simulink model "hiratsuka_dampa_1DOF"  (R2020a)
settings: Solver=ode4  StartTime=0.0  StopTime=10.0  FixedStep=0.002  RelTol=1e-3
values from neighbouring files (symbols this model uses):
  A = 1    [bode_hiratsuka_damper.m]    (also in exp_dampa.m = 0.007; mf_dampa_1DOF.m = 0.003; mf_feedback_relative.m = 0.003; mf_nonlinear_relative.m = 0.01)
  Aor = 0.1*10^-6    (= 1e-07)    [bode_hiratsuka_damper.m]    (also in exp_dampa.m; mf_dampa_1DOF.m; mf_feedback_relative.m; mf_nonlinear_relative.m)
  Ap = (32.50*0.001)^2*pi/4    (= 0.000829576810089)    [bode_hiratsuka_damper.m]    (also in exp_dampa.m; mf_dampa_1DOF.m; mf_feedback_relative.m; mf_nonlinear_relative.m)
  Cor = 0.8    [bode_hiratsuka_damper.m]    (also in exp_dampa.m; mf_dampa_1DOF.m; mf_feedback_relative.m; mf_nonlinear_relative.m)
  Hz = wv(k)    [bode_hiratsuka_damper.m]    (also in exp_dampa.m = 18.8495559215; mf_dampa_1DOF.m = 6.28318530718; mf_feedback_relative.m = 6.28318530718; mf_nonlinear_relative.m = 6.28318530718)
  k1 = 2200    [mf_dampa_1DOF.m]    (also in mf_feedback_relative.m; mf_nonlinear_relative.m; mf_with_P.m; mf_with_Pm.m)
  k2 = 405    [mf_dampa_1DOF.m]    (also in mf_feedback_relative.m; mf_nonlinear_relative.m; mf_with_P.m; mf_with_Pm.m)
  kappa = 1.4    [bode_hiratsuka_damper.m]    (also in exp_dampa.m; mf_dampa_1DOF.m; mf_feedback_relative.m; mf_nonlinear_relative.m)
  m1 = 1.5    [mf_dampa_1DOF.m]    (also in mf_feedback_relative.m; mf_nonlinear_relative.m; mf_with_P.m; mf_with_Pm.m)
  P0 = 101325    [bode_hiratsuka_damper.m]    (also in exp_dampa.m; mf_dampa_1DOF.m; mf_feedback_relative.m; mf_nonlinear_relative.m)
  row0 = 1.1841    [bode_hiratsuka_damper.m]    (also in exp_dampa.m; mf_dampa_1DOF.m; mf_feedback_relative.m; mf_nonlinear_relative.m)
  x0 = 0.05    [bode_hiratsuka_damper.m]    (also in exp_dampa.m = 0.042; mf_dampa_1DOF.m = 0.042; mf_feedback_relative.m = 0.042; mf_nonlinear_relative.m = 0.042)
settings Model: Creator=Peanatsu  LastModifiedBy=Peanatsu

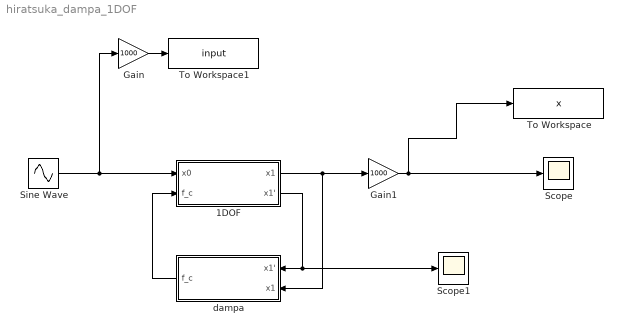
== system hiratsuka_dampa_1DOF ==
  1DOF : Subsystem
  Gain : Gain  Gain=1000
  Gain1 : Gain  Gain=1000
  Scope : Scope
  Scope1 : Scope
  Sine Wave : Sin  Amplitude=A  Frequency=Hz  SampleTime=0
  To Workspace : ToWorkspace  VariableName=x  SaveFormat=Timeseries  SampleTime=-1
  To Workspace1 : ToWorkspace  VariableName=input  SaveFormat=Timeseries  SampleTime=-1
  dampa : Subsystem
  wires:
  1DOF/2(x1') -> Scope1/1, dampa/1(x1')
  1DOF/1(x1) -> Gain1/1, dampa/2(x1)
  dampa/1(f_c) -> 1DOF/2(f_c)
  Sine Wave/1 -> Gain/1, 1DOF/1(x0)
  Gain/1 -> To Workspace1/1
  Gain1/1 -> To Workspace/1, Scope/1

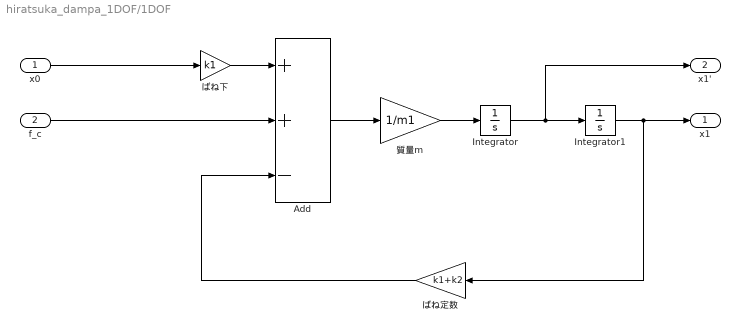
== system hiratsuka_dampa_1DOF/1DOF ==
  x0 : Inport
  f_c : Inport  Port=2
  Add : Sum  Inputs=++-
  Integrator : Integrator
  Integrator1 : Integrator
  ばね下 : Gain  Gain=k1
  "ばね定数 " : Gain  Gain=k1+k2
  質量m : Gain  Gain=1/m1
  x1 : Outport
  x1' : Outport  Port=2
  wires:
  Integrator/1 -> x1'/1, Integrator1/1
  Add/1 -> 質量m/1
  x0/1 -> ばね下/1
  質量m/1 -> Integrator/1
  Integrator1/1 -> x1/1, "ばね定数 "/1
  ばね下/1 -> Add/1
  "ばね定数 "/1 -> Add/3
  f_c/1 -> Add/2

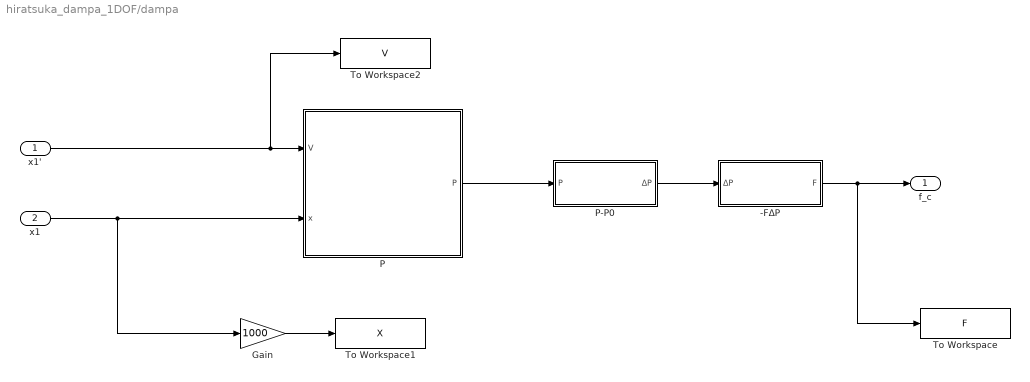
== system hiratsuka_dampa_1DOF/dampa ==
  x1' : Inport
  x1 : Inport  Port=2
  -FΔP : Subsystem
  Gain : Gain  Gain=1000
  P : Subsystem
  P-P0 : Subsystem
  To Workspace : ToWorkspace  VariableName=F  SaveFormat=Timeseries  SampleTime=-1
  To Workspace1 : ToWorkspace  VariableName=X  SaveFormat=Timeseries  SampleTime=-1
  To Workspace2 : ToWorkspace  VariableName=V  SaveFormat=Timeseries  SampleTime=-1
  f_c : Outport
  wires:
  x1'/1 -> To Workspace2/1, P/1(V)
  Gain/1 -> To Workspace1/1
  P/1(P) -> P-P0/1(P)
  P-P0/1(ΔP) -> -FΔP/1(ΔP)
  x1/1 -> P/2(x), Gain/1
  -FΔP/1(F) -> To Workspace/1, f_c/1

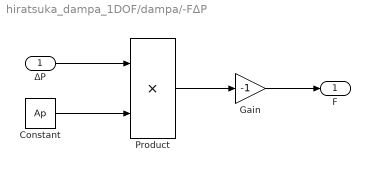
== system hiratsuka_dampa_1DOF/dampa/-FΔP ==
  ΔP : Inport
  Constant : Constant  Value=Ap
  Gain : Gain  Gain=-1
  Product : Product
  F : Outport
  wires:
  Constant/1 -> Product/2
  ΔP/1 -> Product/1
  Product/1 -> Gain/1
  Gain/1 -> F/1

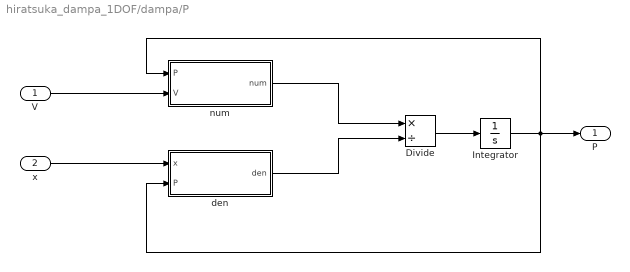
== system hiratsuka_dampa_1DOF/dampa/P ==
  V : Inport
  x : Inport  Port=2
  Divide : Product  Inputs=*/
  Integrator : Integrator  InitialCondition=P0
  den : Subsystem
  num : Subsystem
  P : Outport
  wires:
  Integrator/1 -> P/1, num/1(P), den/2(P)
  V/1 -> num/2(V)
  Divide/1 -> Integrator/1
  x/1 -> den/1(x)
  den/1(den) -> Divide/2
  num/1(num) -> Divide/1

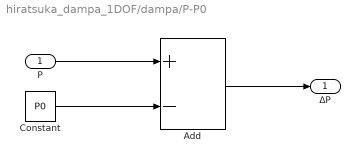
== system hiratsuka_dampa_1DOF/dampa/P-P0 ==
  P : Inport
  Add : Sum  Inputs=+-
  Constant : Constant  Value=P0
  ΔP : Outport
  wires:
  P/1 -> Add/1
  Constant/1 -> Add/2
  Add/1 -> ΔP/1

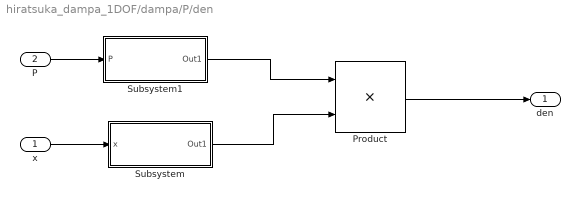
== system hiratsuka_dampa_1DOF/dampa/P/den ==
  x : Inport
  P : Inport  Port=2
  Product : Product
  Subsystem : Subsystem
  Subsystem1 : Subsystem
  den : Outport
  wires:
  x/1 -> Subsystem/1(x)
  P/1 -> Subsystem1/1(P)
  Subsystem1/1(Out1) -> Product/1
  Subsystem/1(Out1) -> Product/2
  Product/1 -> den/1

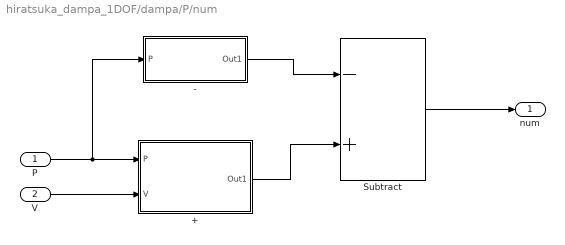
== system hiratsuka_dampa_1DOF/dampa/P/num ==
  P : Inport
  V : Inport  Port=2
  + : Subsystem
  - : Subsystem
  Subtract : Sum  Inputs=-+
  num : Outport
  wires:
  V/1 -> +/2(V)
  P/1 -> -/1(P), +/1(P)
  +/1(Out1) -> Subtract/2
  -/1(Out1) -> Subtract/1
  Subtract/1 -> num/1

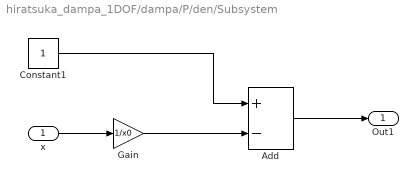
== system hiratsuka_dampa_1DOF/dampa/P/den/Subsystem ==
  x : Inport
  Add : Sum  Inputs=+-
  Constant1 : Constant
  Gain : Gain  Gain=1/x0
  Out1 : Outport
  wires:
  Gain/1 -> Add/2
  Constant1/1 -> Add/1
  Add/1 -> Out1/1
  x/1 -> Gain/1

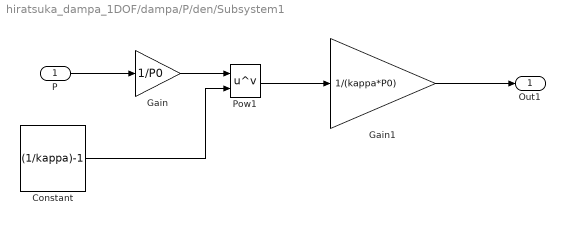
== system hiratsuka_dampa_1DOF/dampa/P/den/Subsystem1 ==
  P : Inport
  Constant : Constant  Value=(1/kappa)-1
  Gain : Gain  Gain=1/P0
  Gain1 : Gain  Gain=1/(kappa*P0)
  Pow1 : Math  Operator=pow  SignedPower=on  OutputSignalType=real  SaturateOnIntegerOverflow=on
  Out1 : Outport
  wires:
  P/1 -> Gain/1
  Gain/1 -> Pow1/1
  Constant/1 -> Pow1/2
  Gain1/1 -> Out1/1
  Pow1/1 -> Gain1/1

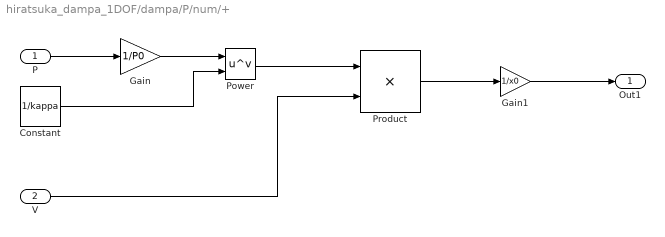
== system hiratsuka_dampa_1DOF/dampa/P/num/+ ==
  P : Inport
  V : Inport  Port=2
  Constant : Constant  Value=1/kappa
  Gain : Gain  Gain=1/P0
  Gain1 : Gain  Gain=1/x0
  Power : Math  Operator=pow  SignedPower=on  OutputSignalType=real  SaturateOnIntegerOverflow=on
  Product : Product
  Out1 : Outport
  wires:
  Gain/1 -> Power/1
  Constant/1 -> Power/2
  Power/1 -> Product/1
  V/1 -> Product/2
  Gain1/1 -> Out1/1
  Product/1 -> Gain1/1
  P/1 -> Gain/1

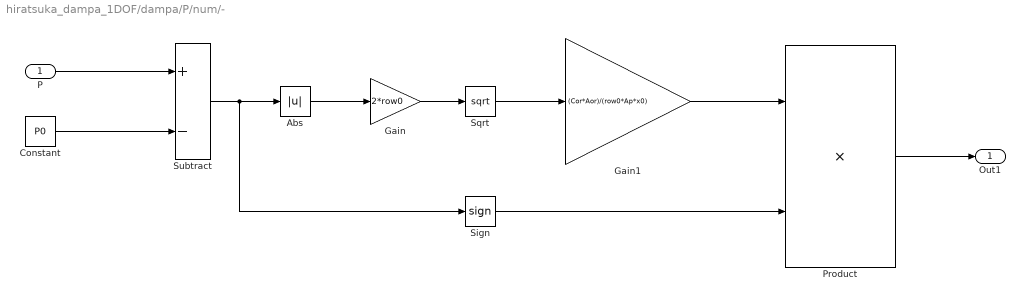
== system hiratsuka_dampa_1DOF/dampa/P/num/- ==
  P : Inport
  Abs : Abs
  Constant : Constant  Value=P0
  Gain : Gain  Gain=2*row0
  Gain1 : Gain  Gain=(Cor*Aor)/(row0*Ap*x0)
  Product : Product
  Sign : Signum
  Sqrt : Sqrt  SaturateOnIntegerOverflow=on
  Subtract : Sum  Inputs=+-
  Out1 : Outport
  wires:
  Abs/1 -> Gain/1
  Gain/1 -> Sqrt/1
  Sqrt/1 -> Gain1/1
  Sign/1 -> Product/2
  Gain1/1 -> Product/1
  Product/1 -> Out1/1
  Subtract/1 -> Sign/1, Abs/1
  P/1 -> Subtract/1
  Constant/1 -> Subtract/2
